simulink model "WTController"  (Simulink 7.5)
settings: Solver=FixedStepDiscrete  StartTime=0.0  StopTime=inf  FixedStep=0.1  RelTol=1e-3
settings Model: Creator=kthwsnt  LastModifiedBy=kthwsn
settings DataIOCC: LimitDataPoints=off  SaveOutput=off  SignalLogging=off  DSMLogging=off  SaveTime=off
settings OptimizationCC: InitFltsAndDblsToZero=on
settings DebuggingCC: StrictBusMsg=Warning

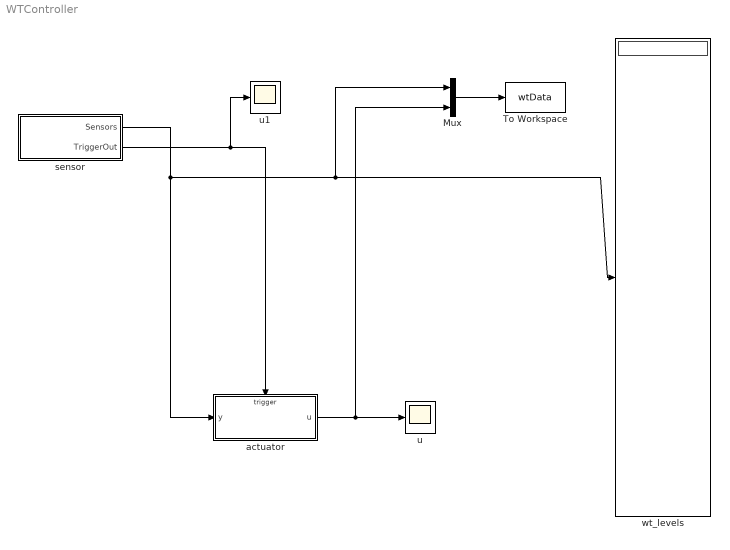
== system WTController ==
  Mux : Mux  Inputs=2
  To Workspace : ToWorkspace  VariableName=wtData  SampleTime=-1  SaveFormat=Structure With Time
  actuator : Subsystem  TreatAsAtomicUnit=on
  sensor : Subsystem  TreatAsAtomicUnit=on
  u : Scope
      settings: YMin=-1  YMax=1
  u1 : Scope
      settings: YMin=0  YMax=1
  wt_levels : Display
  wires:
  sensor/1(Sensors) -> actuator/1(y), wt_levels/1, Mux/1
  sensor/2(TriggerOut) -> actuator/Trigger, u1/1
  actuator/1(u) -> u/1, Mux/2
  Mux/1 -> To Workspace/1

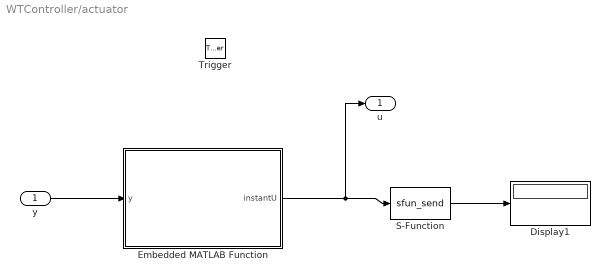
== system WTController/actuator ==
  y : Inport  OutDataType=fixdt(1, 16)  OutScaling=2^0
  Trigger : TriggerPort  TriggerType=either  ShowOutputPort=on
  Display1 : Display
  Embedded MATLAB Function : Stateflow chart  TreatAsAtomicUnit=on
  S-Function : S-Function  FunctionName=sfun_send  SFunctionModules='sfsource'  EnableBusSupport=off
  u : Outport  OutDataType=fixdt(1, 16)  OutScaling=2^0
  wires:
  S-Function/1 -> Display1/1
  Embedded MATLAB Function/1(instantU) -> S-Function/1, u/1
  y/1 -> Embedded MATLAB Function/1(y)

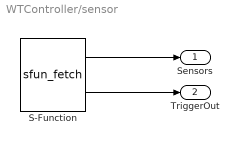
== system WTController/sensor ==
  S-Function : S-Function  FunctionName=sfun_fetch  Parameters=10  SFunctionModules='sfsource'  EnableBusSupport=off
  Sensors : Outport  OutDataType=sfix(16)  OutScaling=2^0
  TriggerOut : Outport  Port=2  OutDataType=sfix(16)  OutScaling=2^0
  wires:
  S-Function/1 -> Sensors/1
  S-Function/2 -> TriggerOut/1

== matlab function actuator/Embedded MATLAB Function ==
  data: instantU output double; y input double
function instantU    = controller(y)

UPDATE_INTERVAL = 20;     % check app_sensors_nbe.h
NUMBER_WT = 10;           % check app_sensors_nbe.h
WT_CALIBRATION = 87.3932; % check app_wt_calibration.h
WT_LIMIT = 5;
persistent y_l1 y_l2 u currentFrame;

if isempty(u)
    y_l1 = zeros(UPDATE_INTERVAL, length(y)/2);
    y_l2 = zeros(UPDATE_INTERVAL, length(y)/2);
    u = ones(UPDATE_INTERVAL, length(y)/2)*2048; % init the control voltages
%     for j=1:size(u,1)
%             u(j,:) = u(j,:)*2^(10)+512*j;
%     end
        currentFrame = 1;
end

%#eml
% the payload is as follows
% payload = [wt1_l1 wt1_l2 wt2_l1 wt2_l2 ..... wtN_l1 wtN_l2]

%% update the values in the matrices
wtId = 1;
for i=1:length(y)   
    if i <= NUMBER_WT
       y_l1(currentFrame, wtId) = y(i)*WT_CALIBRATION;
    else
       y_l2(currentFrame, wtId) = y(i)*WT_CALIBRATION;
    end
    wtId = mod(wtId +1, NUMBER_WT);
    if wtId == 0
        wtId = 1;
    end
end



%% update the u matrix with the new values
if currentFrame == UPDATE_INTERVAL +1
    % cal Jim's code
end

% Security constraints
% for i=1:size(y_l1,2)
%     if y_l1(currentFrame,i) > WT_LIMIT || y_l2(currentFrame,i) > WT_LIMIT
%         u(currentFrame, :) = 0;
%     end
% end

instantU = uint16(u(currentFrame, :));
currentFrame = mod(currentFrame +1 , UPDATE_INTERVAL+1);
if currentFrame == 0
    currentFrame = 1;
end
